simulink model "mtiming"  (Simulink 6.3)
settings: Solver=ode4  StartTime=0.0  StopTime=20.0  FixedStep=0.1  RelTol=1e-3
CloseFcn:
  | rtwprivate ssgencode ModelCloseRequest parameter_test
settings Model: Creator=mwood  LastModifiedBy=mshakeri  ExtModeAutoUpdateStatusClock=off  StrictBusMsg=ErrorLevel1
settings DataIOCC: SignalLoggingName=sigsOut
settings OptimizationCC: InlineParams=on  InlineInvariantSignals=on
settings DebuggingCC: SolverPrmCheckMsg=none
settings HardwareCC: TargetUnknown=on
settings RTWCC: RetainRTWFile=on
settings CodeAppCC: IgnoreCustomStorageClasses=off

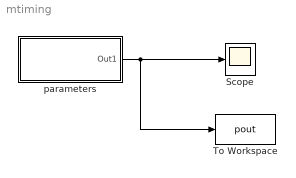
== system mtiming ==
  Scope : Scope
  To Workspace : ToWorkspace  VariableName=pout  SampleTime=-1  SaveFormat=Structure With Time
  parameters : Subsystem  TreatAsAtomicUnit=on
  wires:
  parameters/1(Out1) -> Scope/1, To Workspace/1

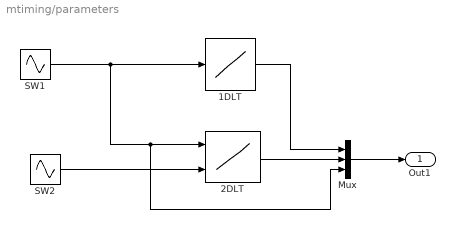
== system mtiming/parameters ==
  1DLT : Lookup  InputValues=[-5:5]  OutputValues=[-5:5]  SaturateOnIntegerOverflow=on
  2DLT : Lookup2D  RowIndex=[-5 0 5]  ColumnIndex=[-9 0 9]  OutputValues=[1 2 3;4 5 6;7 8 9]  SaturateOnIntegerOverflow=on
  Mux : Mux  Inputs=3
  SW1 : Sin  Amplitude=3  Frequency=4  SampleTime=0
  SW2 : Sin  Frequency=3  SampleTime=0
  Out1 : Outport
  wires:
  Mux/1 -> Out1/1
  SW1/1 -> 1DLT/1, 2DLT/1, Mux/3
  1DLT/1 -> Mux/1
  SW2/1 -> 2DLT/2
  2DLT/1 -> Mux/2
